simulink model "model_3"  (R2021b)
settings: Solver=FixedStepAuto  StartTime=0.0  StopTime=10  FixedStep=0.0005  RelTol=1e-3
settings Model: Creator=den  LastModifiedBy=den

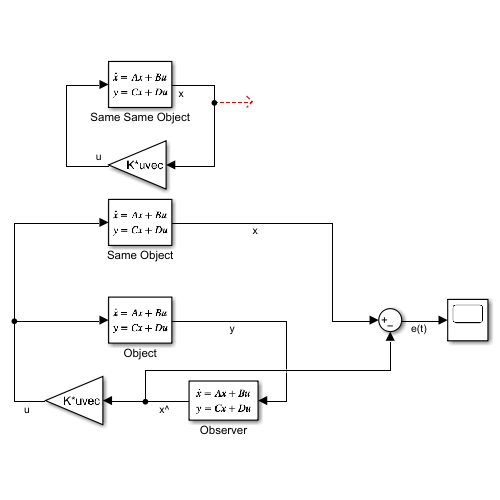
[thumbnail: Simulink's stored preview of the top-level diagram]
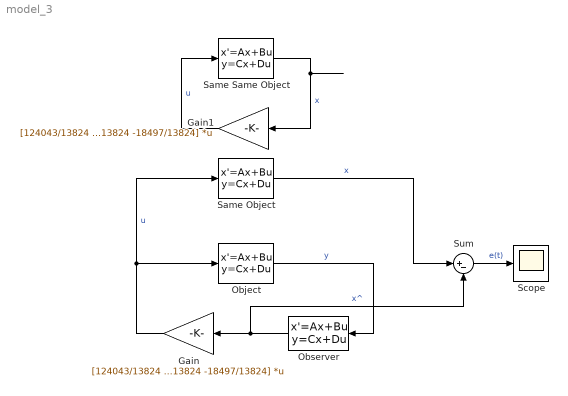
== system model_3 ==
  Gain : Gain  Gain=[124043/13824 -130343/13824 -11357/13824 -18497/13824]  Multiplication=Matrix(K*u) (u vector)
  Gain1 : Gain  Gain=[124043/13824 -130343/13824 -11357/13824 -18497/13824]  Multiplication=Matrix(K*u) (u vector)
  Object : StateSpace  A=[5 -7 -5 1; -7 5 -1 5; -5 -1 5 7; 1 5 7 5]  B=[5; 7; 1; 9]  C=[0 0 2 2; 1 1 -1 1]  D=[0;0]  InitialCondition=[28; -14; 2; -19]
  Observer : StateSpace  A=[55710371/732672 -20493983/732672 12502651/732672 53357815/732672; 19281457/732672 -66303685/732672 -26555911/732672 -68028403/732672; -1420025/732672 -11971795/732672 -1269505/732672 -8844469/732672; 1967405/27136 -7254611/81408 -785537/81408 -2833717/81408]  B=[-11097/424 -11097/424; 37517/1272 37517/1272; 7519/1272 7519/1272; 11773/1272 11773/1272]  C=[1 0 0 0; 0 1 0 0; 0 0 1 0; 0 0 0 1]  D=[0 0; 0 0; 0 0; 0 0]  InitialCondition=[-9;4;32;7]
  Same Object : StateSpace  A=[5 -7 -5 1; -7 5 -1 5; -5 -1 5 7; 1 5 7 5]  B=[5; 7; 1; 9]  C=[1 0 0 0; 0 1 0 0; 0 0 1 0; 0 0 0 1]  D=[0; 0; 0; 0]  InitialCondition=[28; -14; 2; -19]
  Same Same Object : StateSpace  A=[5 -7 -5 1; -7 5 -1 5; -5 -1 5 7; 1 5 7 5]  B=[5; 7; 1; 9]  C=[1 0 0 0; 0 1 0 0; 0 0 1 0; 0 0 0 1]  D=[0; 0; 0; 0]  InitialCondition=[28; -14; 2; -19]
  Scope : Scope
  Sum : Sum  Inputs=|+-
  wires:
  Object/1 -> Observer/1  "y"
  Observer/1 -> Sum/2, Gain/1  "x^"
  Gain/1 -> Same Object/1, Object/1  "u"
  Same Object/1 -> Sum/1  "x"
  Same Same Object/1 -> Gain1/1  "x"
  Gain1/1 -> Same Same Object/1  "u"
  Sum/1 -> Scope/1  "e(t)"
